simulink model "lecture09_model"  (Simulink 7.6)
settings: Solver=ode45  StartTime=0.0  StopTime=10.0  RelTol=1e-3
settings Model: Creator=lum  LastModifiedBy=lum

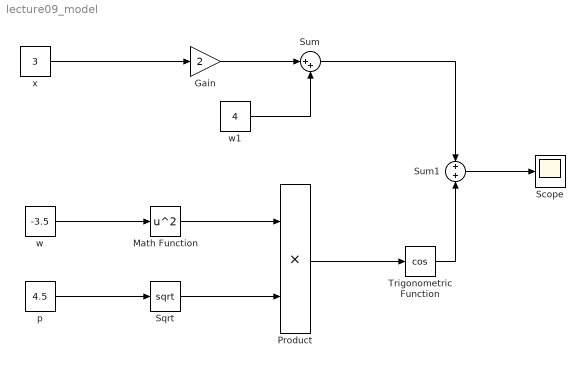
== system lecture09_model ==
  Gain : Gain  Gain=2
  Math Function : Math  Operator=square  SaturateOnIntegerOverflow=on
  Product : Product  RndMeth=Zero
  Scope : Scope
  Sqrt : Sqrt  SaturateOnIntegerOverflow=on
  Sum : Sum  Inputs=|++
  Sum1 : Sum  Inputs=+|+
  Trigonometric Function : Trigonometry  Operator=cos
  p : Constant  Value=4.5
  w : Constant  Value=-3.5
  w1 : Constant  Value=4
  x : Constant  Value=3
  wires:
  x/1 -> Gain/1
  Gain/1 -> Sum/1
  w1/1 -> Sum/2
  Sum/1 -> Sum1/1
  w/1 -> Math Function/1
  p/1 -> Sqrt/1
  Math Function/1 -> Product/1
  Sqrt/1 -> Product/2
  Product/1 -> Trigonometric Function/1
  Trigonometric Function/1 -> Sum1/2
  Sum1/1 -> Scope/1
